simulink model "wlan_mac_dcf_hw"  (Simulink 7.8)
settings: Solver=ode45  StartTime=0.0  StopTime=1e5  RelTol=1e-3
PostLoadFcn:
  | wlan_mac_hw_init
InitFcn:
  | wlan_mac_hw_init
StartFcn:
  | wlan_mac_hw_init
values from neighbouring files (symbols this model uses):
  ticks_per_usec = 10    [wlan_mac_hw_init.m]
undefined symbols (not defined in the file or in its folder): gcbh, xlBlockLoadCallback, xlGetNormalizedPeriod
libraries: xbsIndex_r4 x422, xbsEDKLib_r4 x1
(part 3 of 4)

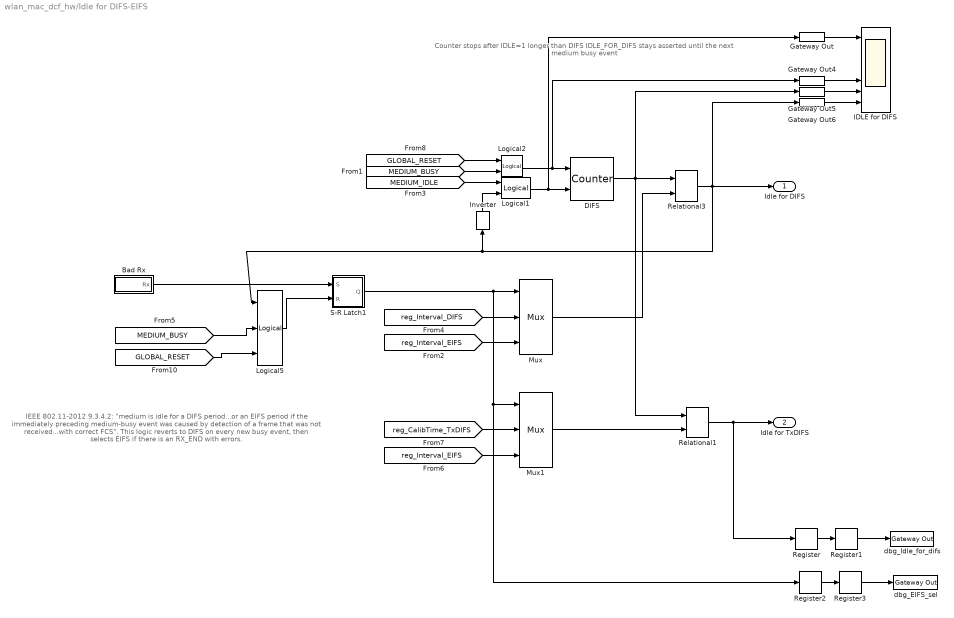
== system wlan_mac_dcf_hw/Idle for DIFS-EIFS ==
  note: IEEE 802.11-2012 9.3.4.2:
      | "medium is idle for a DIFS period...or an EIFS period if the immediately preceding medium-busy
      | event was caused by detection of a frame that was not received...with correct FCS".
      |
      | This logic reverts to DIFS on every new busy event, then
      | selects EIFS if there is an RX_END with errors.
  note: Counter stops after IDLE=1 longer than DIFS
      | IDLE_FOR_DIFS stays asserted until
      | the next medium busy event
  Bad Rx : Subsystem
  DIFS : xbsIndex_r4/Counter  cnt_type=Free Running  cnt_to=inf  operation=Up  start_count=0  cnt_by_val=1  arith_type=Unsigned  n_bits=NB_CNTR_DIFS  bin_pt=0  load_pin=off  rst=on  en=on  explicit_period=off  period=1  dbl_ovrd=off  use_behavioral_HDL=off  implementation=Fabric  block_type=counter
  Gateway Out{,4..6} (4 alike) : xbsIndex_r4/Gateway Out  inherit_from_input=off  hdl_port=off  timing_constraint=None  locs_specified=off  LOCs={}  UseAsDAC=off  DACChannel='1'  block_type=gatewayout
  IDLE for DIFS : Scope  NumInputPorts=7
      settings: YMin=-5~-5~-5~-5~-5~-5~-5  YMax=5~5~5~5~5~5~5  SaveName=ScopeData4
  Inverter : xbsIndex_r4/Inverter  en=off  latency=0  dbl_ovrd=off  block_type=inv
      settings: xl_area=[0 0 0 0 0 0 0]  block_version=VER_STRING_GOES_HERE
  Logical1 : xbsIndex_r4/Logical  logical_function=AND  inputs=2  en=off  latency=0  precision=Full  arith_type=Unsigned  n_bits=16  bin_pt=0  align_bp=on  dbl_ovrd=off  block_type=logical
  Logical2 : xbsIndex_r4/Logical  logical_function=OR  inputs=2  en=off  latency=0  precision=Full  arith_type=Unsigned  n_bits=8  bin_pt=2  align_bp=on  dbl_ovrd=off  block_type=logical
      settings: xl_area=[1 0 0 1 0 0 0]  block_version=VER_STRING_GOES_HERE
  Logical5 : xbsIndex_r4/Logical  logical_function=OR  inputs=3  en=off  latency=0  precision=Full  arith_type=Unsigned  n_bits=16  bin_pt=0  align_bp=on  dbl_ovrd=off  block_type=logical
  Mux : xbsIndex_r4/Mux  inputs=2  en=off  latency=0  precision=Full  arith_type=Unsigned  n_bits=16  bin_pt=14  quantization=Truncate  overflow=Wrap  dbl_ovrd=off  block_type=mux
  Mux1 : xbsIndex_r4/Mux  inputs=2  en=off  latency=0  precision=Full  arith_type=Unsigned  n_bits=16  bin_pt=14  quantization=Truncate  overflow=Wrap  dbl_ovrd=off  block_type=mux
  Register{,1..3} (4 alike) : xbsIndex_r4/Register  init=0  rst=off  en=off  dbl_ovrd=off  block_type=register
  Relational1 : xbsIndex_r4/Relational  mode=a>=b  en=off  latency=0  dbl_ovrd=off  block_type=relational
  Relational3 : xbsIndex_r4/Relational  mode=a>=b  en=off  latency=0  dbl_ovrd=off  block_type=relational
  S-R Latch1 : Subsystem
  dbg_EIFS_sel : xbsIndex_r4/Gateway Out  inherit_from_input=off  hdl_port=on  timing_constraint=None  locs_specified=off  LOCs={}  UseAsDAC=off  DACChannel='1'  block_type=gatewayout
  dbg_Idle_for_difs : xbsIndex_r4/Gateway Out  inherit_from_input=off  hdl_port=on  timing_constraint=None  locs_specified=off  LOCs={}  UseAsDAC=off  DACChannel='1'  block_type=gatewayout
  Idle for DIFS : Outport
  Idle for TxDIFS : Outport  Port=2
  wires:
  Relational3/1 -> Idle for DIFS/1, Inverter/1, Logical5/1, Gateway Out6/1
  Mux/1 -> Relational3/2
  DIFS/1 -> Relational3/1, Relational1/1, Gateway Out5/1
  Logical2/1 -> DIFS/1, Gateway Out4/1
  Logical1/1 -> DIFS/2, Gateway Out/1
  [MEDIUM_IDLE] -> Logical1/1
  [reg_Interval_DIFS] -> Mux/2
  [reg_Interval_EIFS] -> Mux/3
  S-R Latch1/1(Q) -> Mux/1, Mux1/1, Register2/1
  Bad Rx/1(Rx) -> S-R Latch1/1(S)
  Logical5/1 -> S-R Latch1/2(R)
  [MEDIUM_BUSY] -> Logical5/2
  [reg_CalibTime_TxDIFS] -> Mux1/2
  [reg_Interval_EIFS] -> Mux1/3
  Mux1/1 -> Relational1/2
  Relational1/1 -> Idle for TxDIFS/1, Register/1
  Inverter/1 -> Logical1/2
  Gateway Out/1 -> IDLE for DIFS/1
  Gateway Out4/1 -> IDLE for DIFS/5
  Gateway Out5/1 -> IDLE for DIFS/6
  Gateway Out6/1 -> IDLE for DIFS/7
  [GLOBAL_RESET] -> Logical5/3
  [MEDIUM_BUSY] -> Logical2/2
  [GLOBAL_RESET] -> Logical2/1
  Register/1 -> Register1/1
  Register1/1 -> dbg_Idle_for_difs/1
  Register2/1 -> Register3/1
  Register3/1 -> dbg_EIFS_sel/1

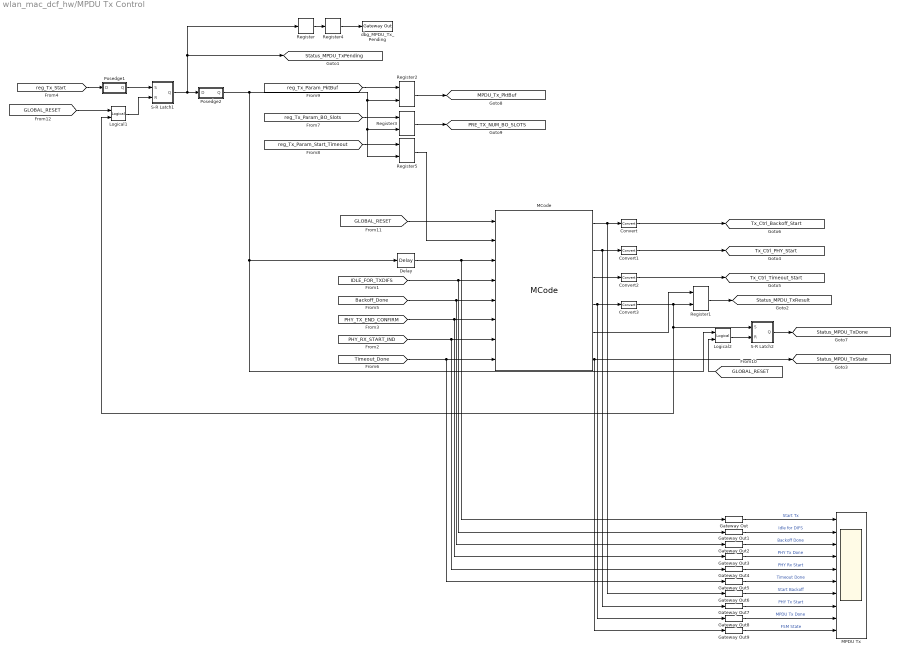
== system wlan_mac_dcf_hw/MPDU Tx Control ==
  Convert{,1..3} (4 alike) : xbsIndex_r4/Convert  gui_display_data_type=Boolean  arith_type=Boolean  n_bits=16  bin_pt=14  float_type=Single  exp_bits=8  fraction_bits=24  quantization=Truncate  overflow=Wrap  en=off  latency=0  dbl_ovrd=off  pipeline=off  block_type=convert
  Delay : xbsIndex_r4/Delay  rst=off  infoeditControl=Selection of Reset will increase slice count due to use of real FFs and instead of SRLs  en=off  latency=1  dbl_ovrd=off  reg_retiming=off  block_type=delay
  Gateway Out{,1..9} (10 alike) : xbsIndex_r4/Gateway Out  inherit_from_input=off  hdl_port=off  timing_constraint=None  locs_specified=off  LOCs={}  UseAsDAC=off  DACChannel='1'  block_type=gatewayout
  Logical1 : xbsIndex_r4/Logical  logical_function=OR  inputs=2  en=off  latency=0  precision=Full  arith_type=Unsigned  n_bits=8  bin_pt=2  align_bp=on  dbl_ovrd=off  block_type=logical
      settings: xl_area=[1 0 0 1 0 0 0]  block_version=VER_STRING_GOES_HERE
  Logical2 : xbsIndex_r4/Logical  logical_function=OR  inputs=2  en=off  latency=0  precision=Full  arith_type=Unsigned  n_bits=8  bin_pt=2  align_bp=on  dbl_ovrd=off  block_type=logical
      settings: xl_area=[1 0 0 1 0 0 0]  block_version=VER_STRING_GOES_HERE
  MCode : xbsIndex_r4/MCode  mfname=mac_tx_ctrl_fsm  explicit_period=on  period=1  inputsTable={'boundInpExpr'=>['','','','','','','',''],'inputs'=>['reset','timeout_req','new_tx','idle_for_difs','backoff_done','phy_tx_done','phy_rx_start','timeout_done']}  outputsTable={'outputs'=>['backoff_start','phy_tx_start','timeout_start','tx_done','tx_result_out','fsm_state_out'],'suppressOut'=>['off','off','off','off','off','off']}  dbl_ovrd=off  enable_stdout=off  enable_debug=off  suppress_output=on  defparams={}  hide_port_list={}  block_type=mcode
  MPDU Tx : Scope  NumInputPorts=10
      settings: YMin=-5~-5~-5~-5~-5~-5~-5~-5~-5~-5  YMax=5~5~5~5~5~5~5~5~5~5
  Posedge1 : Subsystem
  Posedge2 : Subsystem
  Register : xbsIndex_r4/Register  init=0  rst=off  en=off  dbl_ovrd=off  block_type=register
  Register{1..3,5} (4 alike) : xbsIndex_r4/Register  init=0  rst=off  en=on  dbl_ovrd=off  block_type=register
  Register4 : xbsIndex_r4/Register  init=0  rst=off  en=off  dbl_ovrd=off  block_type=register
  S-R Latch1 : Subsystem
  S-R Latch2 : Subsystem
  dbg_MPDU_Tx_Pending : xbsIndex_r4/Gateway Out  inherit_from_input=off  hdl_port=on  timing_constraint=None  locs_specified=off  LOCs={}  UseAsDAC=off  DACChannel='1'  block_type=gatewayout
  tag scope: MPDU_Tx_PktBuf=global, PRE_TX_NUM_BO_SLOTS=global, Status_MPDU_TxDone=global, Status_MPDU_TxPending=global, Status_MPDU_TxResult=global, Status_MPDU_TxState=global, Tx_Ctrl_Backoff_Start=global, Tx_Ctrl_PHY_Start=global, Tx_Ctrl_Timeout_Start=global
  wires:
  [reg_Tx_Param_BO_Slots] -> Register3/1
  [reg_Tx_Start] -> Posedge1/1(D)
  Posedge1/1(Q) -> S-R Latch1/1(S)
  S-R Latch1/1(Q) -> Posedge2/1(D), [Status_MPDU_TxPending], Register/1
  Posedge2/1(Q) -> Register3/2, Register5/2, Register2/2, Delay/1, Logical2/1
  Register3/1 -> [PRE_TX_NUM_BO_SLOTS]
  [reg_Tx_Param_PktBuf] -> Register2/1
  Register2/1 -> [MPDU_Tx_PktBuf]
  [reg_Tx_Param_Start_Timeout] -> Register5/1
  Delay/1 -> MCode/3, Gateway Out/1
  Register5/1 -> MCode/2
  [IDLE_FOR_TXDIFS] -> MCode/4, Gateway Out1/1
  [Backoff_Done] -> MCode/5, Gateway Out2/1
  [PHY_TX_END_CONFIRM] -> MCode/6, Gateway Out3/1
  [PHY_RX_START_IND] -> MCode/7, Gateway Out4/1
  [Timeout_Done] -> MCode/8, Gateway Out5/1
  [GLOBAL_RESET] -> MCode/1
  Logical1/1 -> S-R Latch1/2(R)
  [GLOBAL_RESET] -> Logical1/1
  MCode/4 -> Convert3/1, Gateway Out8/1
  MCode/2 -> Convert1/1, Gateway Out7/1
  MCode/3 -> Convert2/1
  MCode/1 -> Convert/1, Gateway Out6/1
  MCode/5 -> Register1/1
  Register1/1 -> [Status_MPDU_TxResult]
  MCode/6 -> [Status_MPDU_TxState], Gateway Out9/1
  S-R Latch2/1(Q) -> [Status_MPDU_TxDone]
  Convert/1 -> [Tx_Ctrl_Backoff_Start]
  Convert1/1 -> [Tx_Ctrl_PHY_Start]
  Convert2/1 -> [Tx_Ctrl_Timeout_Start]
  Convert3/1 -> Register1/2, S-R Latch2/1(S), Logical1/2
  Logical2/1 -> S-R Latch2/2(R)
  [GLOBAL_RESET] -> Logical2/2
  Gateway Out/1 -> MPDU Tx/1  "Start Tx"
  Gateway Out1/1 -> MPDU Tx/2  "Idle for DIFS"
  Gateway Out2/1 -> MPDU Tx/3  "Backoff Done"
  Gateway Out3/1 -> MPDU Tx/4  "PHY Tx Done"
  Gateway Out4/1 -> MPDU Tx/5  "PHY Rx Start"
  Gateway Out5/1 -> MPDU Tx/6  "Timeout Done"
  Gateway Out6/1 -> MPDU Tx/7  "Start Backoff"
  Gateway Out7/1 -> MPDU Tx/8  "PHY Tx Start"
  Gateway Out8/1 -> MPDU Tx/9  "MPDU Tx Done"
  Gateway Out9/1 -> MPDU Tx/10  "FSM State"
  Register/1 -> Register4/1
  Register4/1 -> dbg_MPDU_Tx_Pending/1

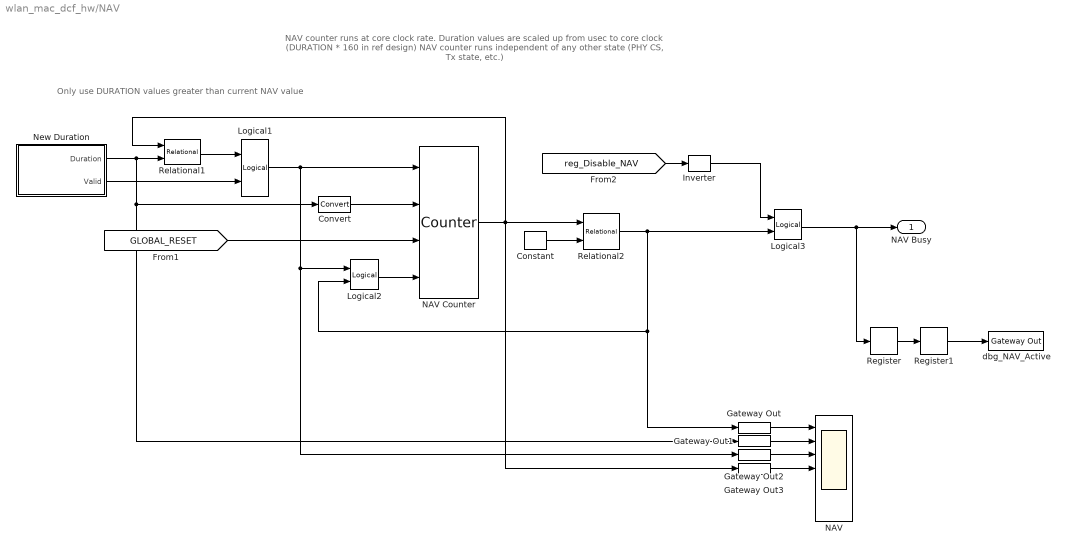
== system wlan_mac_dcf_hw/NAV ==
  note: NAV counter runs at core clock rate. Duration
      | values are scaled up from usec to core clock
      | (DURATION * 160 in ref design)
      |
      | NAV counter runs independent of any
      | other state (PHY CS, Tx state, etc.)
  note: Only use DURATION values greater
      | than current NAV value
  Constant : xbsIndex_r4/Constant  const=0  gui_display_data_type=Fixed-point  arith_type=Unsigned  n_bits=1  bin_pt=0  preci_type=Single  exp_width=8  frac_width=24  explicit_period=off  period=1  equ=P=C  opselect=C  inp2=PCIN>>17  opr=+  inp1=P  carry=CIN  dbl_ovrd=off  block_type=constant
  Convert : xbsIndex_r4/Convert  gui_display_data_type=Fixed-point  arith_type=Unsigned  n_bits=NB_CNTR_NAV  bin_pt=0  float_type=Single  exp_bits=8  fraction_bits=24  quantization=Truncate  overflow=Wrap  en=off  latency=0  dbl_ovrd=off  pipeline=off  block_type=convert
  Gateway Out{,1..3} (4 alike) : xbsIndex_r4/Gateway Out  inherit_from_input=off  hdl_port=off  timing_constraint=None  locs_specified=off  LOCs={}  UseAsDAC=off  DACChannel='1'  block_type=gatewayout
  Inverter : xbsIndex_r4/Inverter  en=off  latency=0  dbl_ovrd=off  block_type=inv
      settings: xl_area=[0 0 0 0 0 0 0]  block_version=VER_STRING_GOES_HERE
  Logical1 : xbsIndex_r4/Logical  logical_function=AND  inputs=2  en=off  latency=0  precision=Full  arith_type=Unsigned  n_bits=16  bin_pt=0  align_bp=on  dbl_ovrd=off  block_type=logical
  Logical2 : xbsIndex_r4/Logical  logical_function=OR  inputs=2  en=off  latency=0  precision=Full  arith_type=Unsigned  n_bits=16  bin_pt=0  align_bp=on  dbl_ovrd=off  block_type=logical
  Logical3 : xbsIndex_r4/Logical  logical_function=AND  inputs=2  en=off  latency=0  precision=Full  arith_type=Unsigned  n_bits=16  bin_pt=0  align_bp=on  dbl_ovrd=off  block_type=logical
  NAV : Scope  NumInputPorts=7
      settings: YMin=-5~-5~-5~-5~-5~-5~-5  YMax=5~5~5~5~5~5~5  SaveName=ScopeData3
  NAV Counter : xbsIndex_r4/Counter  cnt_type=Free Running  cnt_to=Inf  operation=Down  start_count=0  cnt_by_val=1  arith_type=Unsigned  n_bits=NB_CNTR_NAV  bin_pt=0  load_pin=on  rst=on  en=on  explicit_period=on  period=1  dbl_ovrd=off  use_behavioral_HDL=off  implementation=Fabric  block_type=counter
  New Duration : Subsystem
  Register : xbsIndex_r4/Register  init=0  rst=off  en=off  dbl_ovrd=off  block_type=register
  Register1 : xbsIndex_r4/Register  init=0  rst=off  en=off  dbl_ovrd=off  block_type=register
  Relational1 : xbsIndex_r4/Relational  mode=a<b  en=off  latency=0  dbl_ovrd=off  block_type=relational
  Relational2 : xbsIndex_r4/Relational  mode=a>b  en=off  latency=0  dbl_ovrd=off  block_type=relational
  dbg_NAV_Active : xbsIndex_r4/Gateway Out  inherit_from_input=off  hdl_port=on  timing_constraint=None  locs_specified=off  LOCs={}  UseAsDAC=off  DACChannel='1'  block_type=gatewayout
  NAV Busy : Outport
  wires:
  Logical1/1 -> NAV Counter/1, Logical2/1, Gateway Out2/1
  New Duration/2(Valid) -> Logical1/2
  NAV Counter/1 -> Relational2/1, Relational1/1, Gateway Out3/1
  [GLOBAL_RESET] -> NAV Counter/3
  Constant/1 -> Relational2/2
  Relational2/1 -> Gateway Out/1, Logical2/2, Logical3/2
  New Duration/1(Duration) -> Relational1/2, Convert/1, Gateway Out1/1
  Relational1/1 -> Logical1/1
  Convert/1 -> NAV Counter/2
  Gateway Out/1 -> NAV/1
  Gateway Out1/1 -> NAV/2
  Gateway Out2/1 -> NAV/3
  Gateway Out3/1 -> NAV/4
  Logical2/1 -> NAV Counter/4
  Logical3/1 -> NAV Busy/1, Register/1
  [reg_Disable_NAV] -> Inverter/1
  Inverter/1 -> Logical3/1
  Register/1 -> Register1/1
  Register1/1 -> dbg_NAV_Active/1

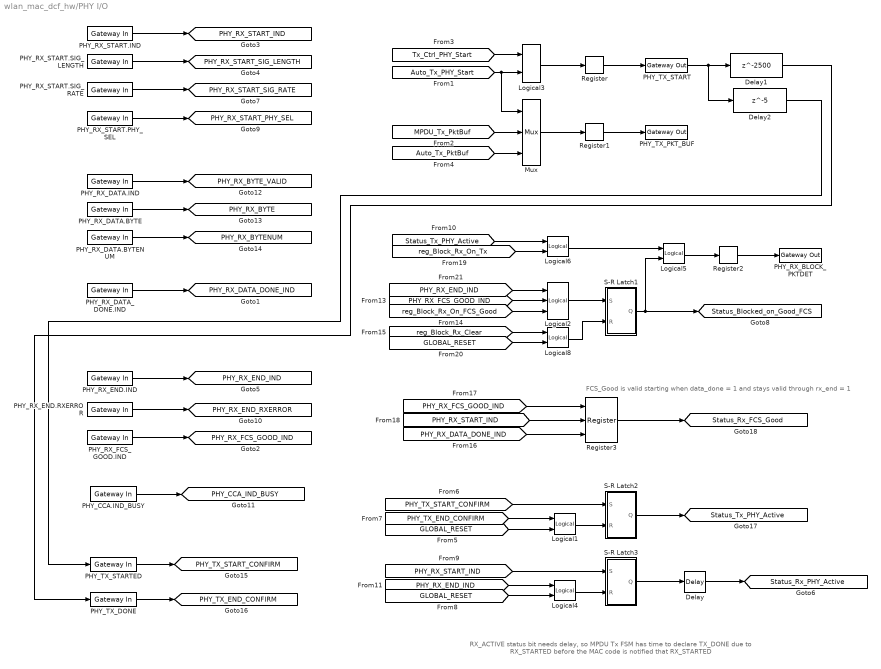
== system wlan_mac_dcf_hw/PHY I/O ==
  note: FCS_Good is valid starting when
      | data_done = 1 and stays valid through
      | rx_end = 1
  note: RX_ACTIVE status bit needs delay, so MPDU Tx FSM has time to declare TX_DONE
      |   due to RX_STARTED before the MAC code is notified that RX_STARTED
  Delay : xbsIndex_r4/Delay  rst=off  infoeditControl=Selection of Reset will increase slice count due to use of real FFs and instead of SRLs  en=off  latency=3  dbl_ovrd=off  reg_retiming=off  block_type=delay
  Delay1 : Delay  DelayLength=2500
  Delay2 : Delay  DelayLength=5
  Logical{1,4..5,8} (4 alike) : xbsIndex_r4/Logical  logical_function=OR  inputs=2  en=off  latency=0  precision=Full  arith_type=Unsigned  n_bits=8  bin_pt=2  align_bp=on  dbl_ovrd=off  block_type=logical
      settings: xl_area=[1 0 0 1 0 0 0]  block_version=VER_STRING_GOES_HERE
  Logical2 : xbsIndex_r4/Logical  logical_function=AND  inputs=3  en=off  latency=0  precision=Full  arith_type=Unsigned  n_bits=8  bin_pt=2  align_bp=on  dbl_ovrd=off  block_type=logical
      settings: xl_area=[1 0 0 1 0 0 0]  block_version=VER_STRING_GOES_HERE
  Logical3 : xbsIndex_r4/Logical  logical_function=OR  inputs=2  en=off  latency=0  precision=Full  arith_type=Unsigned  n_bits=16  bin_pt=0  align_bp=on  dbl_ovrd=off  block_type=logical
  Logical6 : xbsIndex_r4/Logical  logical_function=AND  inputs=2  en=off  latency=0  precision=Full  arith_type=Unsigned  n_bits=8  bin_pt=2  align_bp=on  dbl_ovrd=off  block_type=logical
      settings: xl_area=[1 0 0 1 0 0 0]  block_version=VER_STRING_GOES_HERE
  Mux : xbsIndex_r4/Mux  inputs=2  en=off  latency=0  precision=Full  arith_type=Unsigned  n_bits=16  bin_pt=14  quantization=Truncate  overflow=Wrap  dbl_ovrd=off  block_type=mux
  PHY_CCA.IND_BUSY : xbsIndex_r4/Gateway In  gui_display_data_type=Boolean  arith_type=Boolean  n_bits=16  bin_pt=14  preci_type=Single  exp_width=8  frac_width=24  quantization="Round  (unbiased: +/- Inf)"  overflow=Saturate  period=1  dbl_ovrd=off  timing_constraint=None  locs_specified=off  LOCs={}  UseAsADC=off  ADCChannel='1'  inherit_from_input=off  hdl_port=on  block_type=gatewayin
  PHY_RX_BLOCK_PKTDET : xbsIndex_r4/Gateway Out  inherit_from_input=off  hdl_port=on  timing_constraint=None  locs_specified=off  LOCs={}  UseAsDAC=off  DACChannel='1'  block_type=gatewayout
  PHY_RX_DATA.BYTE : xbsIndex_r4/Gateway In  gui_display_data_type=Fixed-point  arith_type=Unsigned  n_bits=8  bin_pt=0  preci_type=Single  exp_width=8  frac_width=24  quantization="Round  (unbiased: +/- Inf)"  overflow=Saturate  period=1  dbl_ovrd=off  timing_constraint=None  locs_specified=off  LOCs={}  UseAsADC=off  ADCChannel='1'  inherit_from_input=off  hdl_port=on  block_type=gatewayin
  PHY_RX_DATA.BYTENUM : xbsIndex_r4/Gateway In  gui_display_data_type=Fixed-point  arith_type=Unsigned  n_bits=14  bin_pt=0  preci_type=Single  exp_width=8  frac_width=24  quantization="Round  (unbiased: +/- Inf)"  overflow=Saturate  period=1  dbl_ovrd=off  timing_constraint=None  locs_specified=off  LOCs={}  UseAsADC=off  ADCChannel='1'  inherit_from_input=off  hdl_port=on  block_type=gatewayin
  PHY_RX_DATA.IND : xbsIndex_r4/Gateway In  gui_display_data_type=Boolean  arith_type=Boolean  n_bits=16  bin_pt=14  preci_type=Single  exp_width=8  frac_width=24  quantization="Round  (unbiased: +/- Inf)"  overflow=Saturate  period=1  dbl_ovrd=off  timing_constraint=None  locs_specified=off  LOCs={}  UseAsADC=off  ADCChannel='1'  inherit_from_input=off  hdl_port=on  block_type=gatewayin
  PHY_RX_DATA_DONE.IND : xbsIndex_r4/Gateway In  gui_display_data_type=Boolean  arith_type=Boolean  n_bits=1  bin_pt=0  preci_type=Single  exp_width=8  frac_width=24  quantization="Round  (unbiased: +/- Inf)"  overflow=Saturate  period=1  dbl_ovrd=off  timing_constraint=None  locs_specified=off  LOCs={}  UseAsADC=off  ADCChannel='1'  inherit_from_input=off  hdl_port=on  block_type=gatewayin
  PHY_RX_END.IND : xbsIndex_r4/Gateway In  gui_display_data_type=Boolean  arith_type=Boolean  n_bits=16  bin_pt=14  preci_type=Single  exp_width=8  frac_width=24  quantization="Round  (unbiased: +/- Inf)"  overflow=Saturate  period=1  dbl_ovrd=off  timing_constraint=None  locs_specified=off  LOCs={}  UseAsADC=off  ADCChannel='1'  inherit_from_input=off  hdl_port=on  block_type=gatewayin
  PHY_RX_END.RXERROR : xbsIndex_r4/Gateway In  gui_display_data_type=Fixed-point  arith_type=Unsigned  n_bits=2  bin_pt=0  preci_type=Single  exp_width=8  frac_width=24  quantization="Round  (unbiased: +/- Inf)"  overflow=Saturate  period=1  dbl_ovrd=off  timing_constraint=None  locs_specified=off  LOCs={}  UseAsADC=off  ADCChannel='1'  inherit_from_input=off  hdl_port=on  block_type=gatewayin
  PHY_RX_FCS_GOOD.IND : xbsIndex_r4/Gateway In  gui_display_data_type=Boolean  arith_type=Boolean  n_bits=1  bin_pt=0  preci_type=Single  exp_width=8  frac_width=24  quantization="Round  (unbiased: +/- Inf)"  overflow=Saturate  period=1  dbl_ovrd=off  timing_constraint=None  locs_specified=off  LOCs={}  UseAsADC=off  ADCChannel='1'  inherit_from_input=off  hdl_port=on  block_type=gatewayin
  PHY_RX_START.IND : xbsIndex_r4/Gateway In  gui_display_data_type=Boolean  arith_type=Boolean  n_bits=16  bin_pt=14  preci_type=Single  exp_width=8  frac_width=24  quantization="Round  (unbiased: +/- Inf)"  overflow=Saturate  period=1  dbl_ovrd=off  timing_constraint=None  locs_specified=off  LOCs={}  UseAsADC=off  ADCChannel='1'  inherit_from_input=off  hdl_port=on  block_type=gatewayin
  PHY_RX_START.PHY_SEL : xbsIndex_r4/Gateway In  gui_display_data_type=Boolean  arith_type=Boolean  n_bits=16  bin_pt=14  preci_type=Single  exp_width=8  frac_width=24  quantization="Round  (unbiased: +/- Inf)"  overflow=Saturate  period=1  dbl_ovrd=off  timing_constraint=None  locs_specified=off  LOCs={}  UseAsADC=off  ADCChannel='1'  inherit_from_input=off  hdl_port=on  block_type=gatewayin
  PHY_RX_START.SIG_LENGTH : xbsIndex_r4/Gateway In  gui_display_data_type=Fixed-point  arith_type=Unsigned  n_bits=12  bin_pt=0  preci_type=Single  exp_width=8  frac_width=24  quantization="Round  (unbiased: +/- Inf)"  overflow=Saturate  period=1  dbl_ovrd=off  timing_constraint=None  locs_specified=off  LOCs={}  UseAsADC=off  ADCChannel='1'  inherit_from_input=off  hdl_port=on  block_type=gatewayin
  PHY_RX_START.SIG_RATE : xbsIndex_r4/Gateway In  gui_display_data_type=Fixed-point  arith_type=Unsigned  n_bits=4  bin_pt=0  preci_type=Single  exp_width=8  frac_width=24  quantization="Round  (unbiased: +/- Inf)"  overflow=Saturate  period=1  dbl_ovrd=off  timing_constraint=None  locs_specified=off  LOCs={}  UseAsADC=off  ADCChannel='1'  inherit_from_input=off  hdl_port=on  block_type=gatewayin
  PHY_TX_DONE : xbsIndex_r4/Gateway In  gui_display_data_type=Boolean  arith_type=Boolean  n_bits=16  bin_pt=14  preci_type=Single  exp_width=8  frac_width=24  quantization="Round  (unbiased: +/- Inf)"  overflow=Saturate  period=1  dbl_ovrd=off  timing_constraint=None  locs_specified=off  LOCs={}  UseAsADC=off  ADCChannel='1'  inherit_from_input=off  hdl_port=on  block_type=gatewayin
  PHY_TX_PKT_BUF : xbsIndex_r4/Gateway Out  inherit_from_input=off  hdl_port=on  timing_constraint=None  locs_specified=off  LOCs={}  UseAsDAC=off  DACChannel='1'  block_type=gatewayout
  PHY_TX_START : xbsIndex_r4/Gateway Out  inherit_from_input=off  hdl_port=on  timing_constraint=None  locs_specified=off  LOCs={}  UseAsDAC=off  DACChannel='1'  block_type=gatewayout
  PHY_TX_STARTED : xbsIndex_r4/Gateway In  gui_display_data_type=Boolean  arith_type=Boolean  n_bits=16  bin_pt=14  preci_type=Single  exp_width=8  frac_width=24  quantization="Round  (unbiased: +/- Inf)"  overflow=Saturate  period=1  dbl_ovrd=off  timing_constraint=None  locs_specified=off  LOCs={}  UseAsADC=off  ADCChannel='1'  inherit_from_input=off  hdl_port=on  block_type=gatewayin
  Register : xbsIndex_r4/Register  init=0  rst=off  en=off  dbl_ovrd=off  block_type=register
  Register1 : xbsIndex_r4/Register  init=0  rst=off  en=off  dbl_ovrd=off  block_type=register
  Register2 : xbsIndex_r4/Register  init=0  rst=off  en=off  dbl_ovrd=off  block_type=register
  Register3 : xbsIndex_r4/Register  init=0  rst=on  en=on  dbl_ovrd=off  block_type=register
  S-R Latch1 : Subsystem
  S-R Latch2 : Subsystem
  S-R Latch3 : Subsystem
  tag scope: PHY_CCA_IND_BUSY=global, PHY_RX_BYTE=global, PHY_RX_BYTENUM=global, PHY_RX_BYTE_VALID=global, PHY_RX_DATA_DONE_IND=global, PHY_RX_END_IND=global, PHY_RX_END_RXERROR=global, PHY_RX_FCS_GOOD_IND=global, PHY_RX_START_IND=global, PHY_RX_START_PHY_SEL=global, PHY_RX_START_SIG_LENGTH=global, PHY_RX_START_SIG_RATE=global, PHY_TX_END_CONFIRM=global, PHY_TX_START_CONFIRM=global, Status_Blocked_on_Good_FCS=global, Status_Rx_FCS_Good=global, Status_Rx_PHY_Active=global, Status_Tx_PHY_Active=global
  wires:
  PHY_RX_DATA_DONE.IND/1 -> [PHY_RX_DATA_DONE_IND]
  PHY_RX_FCS_GOOD.IND/1 -> [PHY_RX_FCS_GOOD_IND]
  PHY_RX_START.IND/1 -> [PHY_RX_START_IND]
  PHY_RX_START.SIG_LENGTH/1 -> [PHY_RX_START_SIG_LENGTH]
  PHY_RX_END.IND/1 -> [PHY_RX_END_IND]
  PHY_RX_END.RXERROR/1 -> [PHY_RX_END_RXERROR]
  PHY_CCA.IND_BUSY/1 -> [PHY_CCA_IND_BUSY]
  PHY_RX_DATA.IND/1 -> [PHY_RX_BYTE_VALID]
  PHY_RX_DATA.BYTE/1 -> [PHY_RX_BYTE]
  PHY_RX_DATA.BYTENUM/1 -> [PHY_RX_BYTENUM]
  PHY_TX_STARTED/1 -> [PHY_TX_START_CONFIRM]
  PHY_TX_DONE/1 -> [PHY_TX_END_CONFIRM]
  Logical3/1 -> Register/1
  [Tx_Ctrl_PHY_Start] -> Logical3/1
  [Auto_Tx_PHY_Start] -> Logical3/2, Mux/1
  Mux/1 -> Register1/1
  [MPDU_Tx_PktBuf] -> Mux/2
  [Auto_Tx_PktBuf] -> Mux/3
  Register/1 -> PHY_TX_START/1
  Register1/1 -> PHY_TX_PKT_BUF/1
  [PHY_TX_START_CONFIRM] -> S-R Latch2/1(S)
  Logical1/1 -> S-R Latch2/2(R)
  [PHY_TX_END_CONFIRM] -> Logical1/1
  [GLOBAL_RESET] -> Logical1/2
  S-R Latch2/1(Q) -> [Status_Tx_PHY_Active]
  [PHY_RX_START_IND] -> S-R Latch3/1(S)
  Logical4/1 -> S-R Latch3/2(R)
  [PHY_RX_END_IND] -> Logical4/1
  [GLOBAL_RESET] -> Logical4/2
  S-R Latch3/1(Q) -> Delay/1
  Register2/1 -> PHY_RX_BLOCK_PKTDET/1
  Logical6/1 -> Logical5/1
  [PHY_RX_END_IND] -> Logical2/1
  [PHY_RX_FCS_GOOD_IND] -> Logical2/2
  [reg_Block_Rx_On_FCS_Good] -> Logical2/3
  Logical2/1 -> S-R Latch1/1(S)
  S-R Latch1/1(Q) -> Logical5/2, [Status_Blocked_on_Good_FCS]
  Logical5/1 -> Register2/1
  PHY_RX_START.SIG_RATE/1 -> [PHY_RX_START_SIG_RATE]
  PHY_RX_START.PHY_SEL/1 -> [PHY_RX_START_PHY_SEL]
  Logical8/1 -> S-R Latch1/2(R)
  [reg_Block_Rx_Clear] -> Logical8/1
  [GLOBAL_RESET] -> Logical8/2
  [PHY_RX_FCS_GOOD_IND] -> Register3/1
  Register3/1 -> [Status_Rx_FCS_Good]
  [PHY_RX_DATA_DONE_IND] -> Register3/3
  [PHY_RX_START_IND] -> Register3/2
  [Status_Tx_PHY_Active] -> Logical6/1
  [reg_Block_Rx_On_Tx] -> Logical6/2
  Delay/1 -> [Status_Rx_PHY_Active]
  PHY_TX_START/1 -> Delay1/1, Delay2/1
  Delay1/1 -> PHY_TX_DONE/1
  Delay2/1 -> PHY_TX_STARTED/1

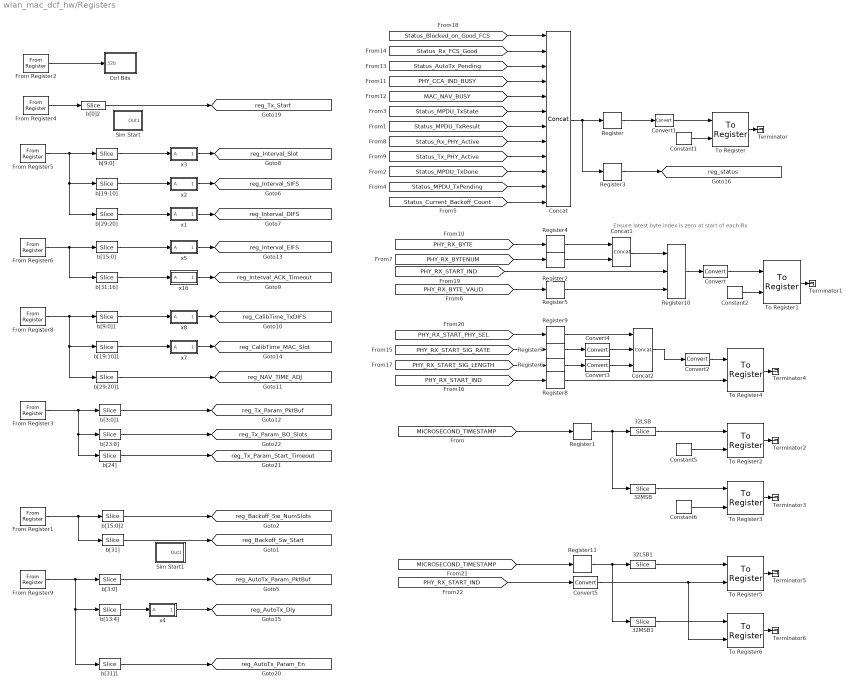
== system wlan_mac_dcf_hw/Registers ==
  note: Ensure latest byte index is zero
      | at start of each Rx
  " b[13:4]" : xbsIndex_r4/Slice  nbits=10  boolean_output=off  mode=Lower Bit Location + Width  bit1=0  base1=MSB of Input  bit0=4  base0=LSB of Input  dbl_ovrd=off  block_type=slice
      settings: block_version=VER_STRING_GOES_HERE
  " b[15:0]" : xbsIndex_r4/Slice  nbits=16  boolean_output=off  mode=Lower Bit Location + Width  bit1=0  base1=MSB of Input  bit0=0  base0=LSB of Input  dbl_ovrd=off  block_type=slice
      settings: block_version=VER_STRING_GOES_HERE
  " b[15:0]2" : xbsIndex_r4/Slice  nbits=16  boolean_output=off  mode=Lower Bit Location + Width  bit1=0  base1=MSB of Input  bit0=0  base0=LSB of Input  dbl_ovrd=off  block_type=slice
      settings: block_version=VER_STRING_GOES_HERE
  " b[19:10]" : xbsIndex_r4/Slice  nbits=10  boolean_output=off  mode=Lower Bit Location + Width  bit1=0  base1=MSB of Input  bit0=10  base0=LSB of Input  dbl_ovrd=off  block_type=slice
      settings: block_version=VER_STRING_GOES_HERE
  " b[19:10]1" : xbsIndex_r4/Slice  nbits=10  boolean_output=off  mode=Lower Bit Location + Width  bit1=0  base1=MSB of Input  bit0=10  base0=LSB of Input  dbl_ovrd=off  block_type=slice
      settings: block_version=VER_STRING_GOES_HERE
  " b[23:8]" : xbsIndex_r4/Slice  nbits=16  boolean_output=off  mode=Lower Bit Location + Width  bit1=0  base1=MSB of Input  bit0=8  base0=LSB of Input  dbl_ovrd=off  block_type=slice
      settings: block_version=VER_STRING_GOES_HERE
  " b[24]" : xbsIndex_r4/Slice  nbits=1  boolean_output=on  mode=Lower Bit Location + Width  bit1=0  base1=MSB of Input  bit0=24  base0=LSB of Input  dbl_ovrd=off  block_type=slice
      settings: block_version=VER_STRING_GOES_HERE
  " b[29:20]" : xbsIndex_r4/Slice  nbits=10  boolean_output=off  mode=Lower Bit Location + Width  bit1=0  base1=MSB of Input  bit0=20  base0=LSB of Input  dbl_ovrd=off  block_type=slice
      settings: block_version=VER_STRING_GOES_HERE
  " b[29:20]1" : xbsIndex_r4/Slice  nbits=10  boolean_output=off  mode=Lower Bit Location + Width  bit1=0  base1=MSB of Input  bit0=20  base0=LSB of Input  dbl_ovrd=off  block_type=slice
      settings: block_version=VER_STRING_GOES_HERE
  " b[31:16]" : xbsIndex_r4/Slice  nbits=16  boolean_output=off  mode=Lower Bit Location + Width  bit1=0  base1=MSB of Input  bit0=16  base0=LSB of Input  dbl_ovrd=off  block_type=slice
      settings: block_version=VER_STRING_GOES_HERE
  " b[31]" : xbsIndex_r4/Slice  nbits=1  boolean_output=on  mode=Lower Bit Location + Width  bit1=0  base1=MSB of Input  bit0=31  base0=LSB of Input  dbl_ovrd=off  block_type=slice
      settings: block_version=VER_STRING_GOES_HERE
  " b[31]1" : xbsIndex_r4/Slice  nbits=1  boolean_output=on  mode=Lower Bit Location + Width  bit1=0  base1=MSB of Input  bit0=31  base0=LSB of Input  dbl_ovrd=off  block_type=slice
      settings: block_version=VER_STRING_GOES_HERE
  " b[3:0]" : xbsIndex_r4/Slice  nbits=4  boolean_output=off  mode=Lower Bit Location + Width  bit1=0  base1=MSB of Input  bit0=0  base0=LSB of Input  dbl_ovrd=off  block_type=slice
      settings: block_version=VER_STRING_GOES_HERE
  " b[3:0]1" : xbsIndex_r4/Slice  nbits=4  boolean_output=off  mode=Lower Bit Location + Width  bit1=0  base1=MSB of Input  bit0=0  base0=LSB of Input  dbl_ovrd=off  block_type=slice
      settings: block_version=VER_STRING_GOES_HERE
  " b[9:0]" : xbsIndex_r4/Slice  nbits=10  boolean_output=off  mode=Lower Bit Location + Width  bit1=0  base1=MSB of Input  bit0=0  base0=LSB of Input  dbl_ovrd=off  block_type=slice
      settings: block_version=VER_STRING_GOES_HERE
  " b[9:0]1" : xbsIndex_r4/Slice  nbits=10  boolean_output=off  mode=Lower Bit Location + Width  bit1=0  base1=MSB of Input  bit0=0  base0=LSB of Input  dbl_ovrd=off  block_type=slice
      settings: block_version=VER_STRING_GOES_HERE
  32LSB : xbsIndex_r4/Slice  nbits=32  boolean_output=off  mode=Lower Bit Location + Width  bit1=0  base1=MSB of Input  bit0=0  base0=LSB of Input  dbl_ovrd=off  block_type=slice
      settings: block_version=VER_STRING_GOES_HERE
  32LSB1 : xbsIndex_r4/Slice  nbits=32  boolean_output=off  mode=Lower Bit Location + Width  bit1=0  base1=MSB of Input  bit0=0  base0=LSB of Input  dbl_ovrd=off  block_type=slice
      settings: block_version=VER_STRING_GOES_HERE
  32MSB : xbsIndex_r4/Slice  nbits=32  boolean_output=off  mode=Upper Bit Location + Width  bit1=0  base1=MSB of Input  bit0=0  base0=LSB of Input  dbl_ovrd=off  block_type=slice
      settings: block_version=VER_STRING_GOES_HERE
  32MSB1 : xbsIndex_r4/Slice  nbits=32  boolean_output=off  mode=Upper Bit Location + Width  bit1=0  base1=MSB of Input  bit0=0  base0=LSB of Input  dbl_ovrd=off  block_type=slice
      settings: block_version=VER_STRING_GOES_HERE
  Concat : xbsIndex_r4/Concat  num_inputs=12  dbl_ovrd=off  block_type=concat
      settings: block_version=8.2.02
  Concat1 : xbsIndex_r4/Concat  num_inputs=2  dbl_ovrd=off  block_type=concat
      settings: block_version=8.2.02
  Concat2 : xbsIndex_r4/Concat  num_inputs=3  dbl_ovrd=off  block_type=concat
      settings: block_version=8.2.02
  Constant{1..2,5..6} (4 alike) : xbsIndex_r4/Constant  const=1  gui_display_data_type=Boolean  arith_type=Boolean  n_bits=30  bin_pt=0  preci_type=Single  exp_width=8  frac_width=24  explicit_period=on  period=1  equ=P=C  opselect=C  inp2=PCIN>>17  opr=+  inp1=P  carry=CIN  dbl_ovrd=off  block_type=constant
  Convert : xbsIndex_r4/Convert  gui_display_data_type=Fixed-point  arith_type=Unsigned  n_bits=32  bin_pt=0  float_type=Single  exp_bits=8  fraction_bits=24  quantization=Truncate  overflow=Wrap  en=off  latency=0  dbl_ovrd=off  pipeline=off  block_type=convert
  Convert1 : xbsIndex_r4/Convert  gui_display_data_type=Fixed-point  arith_type=Unsigned  n_bits=32  bin_pt=0  float_type=Single  exp_bits=8  fraction_bits=24  quantization=Truncate  overflow=Wrap  en=off  latency=0  dbl_ovrd=off  pipeline=off  block_type=convert
  Convert2 : xbsIndex_r4/Convert  gui_display_data_type=Fixed-point  arith_type=Unsigned  n_bits=32  bin_pt=0  float_type=Single  exp_bits=8  fraction_bits=24  quantization=Truncate  overflow=Wrap  en=off  latency=0  dbl_ovrd=off  pipeline=off  block_type=convert
  Convert3 : xbsIndex_r4/Convert  gui_display_data_type=Fixed-point  arith_type=Unsigned  n_bits=16  bin_pt=0  float_type=Single  exp_bits=8  fraction_bits=24  quantization=Truncate  overflow=Wrap  en=off  latency=0  dbl_ovrd=off  pipeline=off  block_type=convert
  Convert4 : xbsIndex_r4/Convert  gui_display_data_type=Fixed-point  arith_type=Unsigned  n_bits=8  bin_pt=0  float_type=Single  exp_bits=8  fraction_bits=24  quantization=Truncate  overflow=Wrap  en=off  latency=0  dbl_ovrd=off  pipeline=off  block_type=convert
  Convert5 : xbsIndex_r4/Convert  gui_display_data_type=Boolean  arith_type=Boolean  n_bits=32  bin_pt=0  float_type=Single  exp_bits=8  fraction_bits=24  quantization=Truncate  overflow=Wrap  en=off  latency=0  dbl_ovrd=off  pipeline=off  block_type=convert
  Ctrl Bits : Subsystem
  From Register1 : xbsIndex_r4/From Register  shared_memory_name='BACKOFF_CTRL'  init=REG_MAC_Backoff_Control  period=1  ownership=Locally owned and initialized  gui_display_data_type=Fixed-point  arith_type=Unsigned  n_bits=32  bin_pt=0  preci_type=Single  dbl_ovrd=off  block_type=fromreg
      settings: AttributesFormatString=<< %<shared_memory_name> >>  infoedit="Register block that reads data to a shared memory register.  Delay of one sample period."
  From Register2 : xbsIndex_r4/From Register  shared_memory_name='Control'  init=0  period=1  ownership=Locally owned and initialized  gui_display_data_type=Fixed-point  arith_type=Unsigned  n_bits=32  bin_pt=0  preci_type=Single  dbl_ovrd=off  block_type=fromreg
      settings: AttributesFormatString=<< %<shared_memory_name> >>  infoedit="Register block that reads data to a shared memory register.  Delay of one sample period."
  From Register3 : xbsIndex_r4/From Register  shared_memory_name='MPDU_TX_PARAMS'  init=REG_MAC_MPDU_Tx_Params  period=1  ownership=Locally owned and initialized  gui_display_data_type=Fixed-point  arith_type=Unsigned  n_bits=32  bin_pt=0  preci_type=Single  dbl_ovrd=off  block_type=fromreg
      settings: AttributesFormatString=<< %<shared_memory_name> >>  infoedit="Register block that reads data to a shared memory register.  Delay of one sample period."
  From Register4 : xbsIndex_r4/From Register  shared_memory_name='TX_START'  init=0  period=1  ownership=Locally owned and initialized  gui_display_data_type=Fixed-point  arith_type=Unsigned  n_bits=32  bin_pt=0  preci_type=Single  dbl_ovrd=off  block_type=fromreg
      settings: AttributesFormatString=<< %<shared_memory_name> >>  infoedit="Register block that reads data to a shared memory register.  Delay of one sample period."
  From Register5 : xbsIndex_r4/From Register  shared_memory_name='IFS_INTERVALS1'  init=REG_MAC_Intervals_1  period=1  ownership=Locally owned and initialized  gui_display_data_type=Fixed-point  arith_type=Unsigned  n_bits=32  bin_pt=0  preci_type=Single  dbl_ovrd=off  block_type=fromreg
      settings: AttributesFormatString=<< %<shared_memory_name> >>  infoedit="Register block that reads data to a shared memory register.  Delay of one sample period."
  From Register6 : xbsIndex_r4/From Register  shared_memory_name='IFS_INTERVALS2'  init=REG_MAC_Intervals_2  period=1  ownership=Locally owned and initialized  gui_display_data_type=Fixed-point  arith_type=Unsigned  n_bits=32  bin_pt=0  preci_type=Single  dbl_ovrd=off  block_type=fromreg
      settings: AttributesFormatString=<< %<shared_memory_name> >>  infoedit="Register block that reads data to a shared memory register.  Delay of one sample period."
  From Register8 : xbsIndex_r4/From Register  shared_memory_name='CALIB_TIMES'  init=REG_MAC_Calib_Times  period=1  ownership=Locally owned and initialized  gui_display_data_type=Fixed-point  arith_type=Unsigned  n_bits=32  bin_pt=0  preci_type=Single  dbl_ovrd=off  block_type=fromreg
      settings: AttributesFormatString=<< %<shared_memory_name> >>  infoedit="Register block that reads data to a shared memory register.  Delay of one sample period."
  From Register9 : xbsIndex_r4/From Register  shared_memory_name='AUTO_TX_PARAMS'  init=REG_MAC_Auto_Tx_Params  period=1  ownership=Locally owned and initialized  gui_display_data_type=Fixed-point  arith_type=Unsigned  n_bits=32  bin_pt=0  preci_type=Single  dbl_ovrd=off  block_type=fromreg
      settings: AttributesFormatString=<< %<shared_memory_name> >>  infoedit="Register block that reads data to a shared memory register.  Delay of one sample period."
  Register{,1..9,11} (11 alike) : xbsIndex_r4/Register  init=0  rst=off  en=off  dbl_ovrd=off  block_type=register
  Register10 : xbsIndex_r4/Register  init=0  rst=on  en=on  dbl_ovrd=off  block_type=register
  Sim Start : Subsystem
  Sim Start1 : Subsystem
  Terminator{,1..6} (7 alike) : Terminator
  To Register : xbsIndex_r4/To Register  shared_memory_name='Status'  init=0  ownership=Locally owned and initialized  explicit_data_type=on  gui_display_data_type=Fixed-point  arith_type=Unsigned  n_bits=32  bin_pt=0  preci_type=Single  dbl_ovrd=off  block_type=toreg
      settings: AttributesFormatString=<< %<shared_memory_name> >>  infoedit="Register block that writes data to a shared memory register.  Delay of one sample period."
  To Register1 : xbsIndex_r4/To Register  shared_memory_name='LATEST_RX_BYTE'  init=0  ownership=Locally owned and initialized  explicit_data_type=on  gui_display_data_type=Fixed-point  arith_type=Unsigned  n_bits=32  bin_pt=0  preci_type=Single  dbl_ovrd=off  block_type=toreg
      settings: AttributesFormatString=<< %<shared_memory_name> >>  infoedit="Register block that writes data to a shared memory register.  Delay of one sample period."
  To Register2 : xbsIndex_r4/To Register  shared_memory_name='TIMESTAMP_LSB'  init=0  ownership=Locally owned and initialized  explicit_data_type=on  gui_display_data_type=Fixed-point  arith_type=Unsigned  n_bits=32  bin_pt=0  preci_type=Single  dbl_ovrd=off  block_type=toreg
      settings: AttributesFormatString=<< %<shared_memory_name> >>  infoedit="Register block that writes data to a shared memory register.  Delay of one sample period."
  To Register3 : xbsIndex_r4/To Register  shared_memory_name='TIMESTAMP_MSB'  init=0  ownership=Locally owned and initialized  explicit_data_type=on  gui_display_data_type=Fixed-point  arith_type=Unsigned  n_bits=32  bin_pt=0  preci_type=Single  dbl_ovrd=off  block_type=toreg
      settings: AttributesFormatString=<< %<shared_memory_name> >>  infoedit="Register block that writes data to a shared memory register.  Delay of one sample period."
  To Register4 : xbsIndex_r4/To Register  shared_memory_name='RX_RATE_LENGTH'  init=0  ownership=Locally owned and initialized  explicit_data_type=on  gui_display_data_type=Fixed-point  arith_type=Unsigned  n_bits=32  bin_pt=0  preci_type=Single  dbl_ovrd=off  block_type=toreg
      settings: AttributesFormatString=<< %<shared_memory_name> >>  infoedit="Register block that writes data to a shared memory register.  Delay of one sample period."
  To Register5 : xbsIndex_r4/To Register  shared_memory_name='RX_START_TIMESTAMP_LSB'  init=0  ownership=Locally owned and initialized  explicit_data_type=on  gui_display_data_type=Fixed-point  arith_type=Unsigned  n_bits=32  bin_pt=0  preci_type=Single  dbl_ovrd=off  block_type=toreg
      settings: AttributesFormatString=<< %<shared_memory_name> >>  infoedit="Register block that writes data to a shared memory register.  Delay of one sample period."
  To Register6 : xbsIndex_r4/To Register  shared_memory_name='RX_START_TIMESTAMP_MSB'  init=0  ownership=Locally owned and initialized  explicit_data_type=on  gui_display_data_type=Fixed-point  arith_type=Unsigned  n_bits=32  bin_pt=0  preci_type=Single  dbl_ovrd=off  block_type=toreg
      settings: AttributesFormatString=<< %<shared_memory_name> >>  infoedit="Register block that writes data to a shared memory register.  Delay of one sample period."
  b[0]2 : xbsIndex_r4/Slice  nbits=1  boolean_output=on  mode=Lower Bit Location + Width  bit1=0  base1=MSB of Input  bit0=0  base0=LSB of Input  dbl_ovrd=off  block_type=slice
      settings: block_version=VER_STRING_GOES_HERE
  x1 : Subsystem
  x16 : Subsystem
  x2 : Subsystem
  x3 : Subsystem
  x4 : Subsystem
  x5 : Subsystem
  x7 : Subsystem
  x8 : Subsystem
  tag scope: reg_AutoTx_Dly=global, reg_AutoTx_Param_En=global, reg_AutoTx_Param_PktBuf=global, reg_Backoff_Sw_NumSlots=global, reg_Backoff_Sw_Start=global, reg_CalibTime_MAC_Slot=global, reg_CalibTime_TxDIFS=global, reg_Interval_ACK_Timeout=global, reg_Interval_DIFS=global, reg_Interval_EIFS=global, reg_Interval_SIFS=global, reg_Interval_Slot=global, reg_NAV_TIME_ADJ=global, reg_Tx_Param_BO_Slots=global, reg_Tx_Param_PktBuf=global, reg_Tx_Param_Start_Timeout=global, reg_Tx_Start=global, reg_status=global
  wires:
  From Register2/1 -> Ctrl Bits/1(32b)
  Constant1/1 -> To Register/2
  To Register/1 -> Terminator/1
  Concat/1 -> Register3/1, Register/1
  32LSB/1 -> To Register2/1
  Constant5/1 -> To Register2/2
  32MSB/1 -> To Register3/1
  Constant6/1 -> To Register3/2
  [MICROSECOND_TIMESTAMP] -> Register1/1
  x16/1(Ax16) -> [reg_Interval_ACK_Timeout]
  x1/1(Ax16) -> [reg_Interval_DIFS]
  x2/1(Ax16) -> [reg_Interval_SIFS]
  x3/1(Ax16) -> [reg_Interval_Slot]
  x5/1(Ax16) -> [reg_Interval_EIFS]
  From Register3/1 -> " b[23:8]"/1, " b[24]"/1, " b[3:0]1"/1
  b[0]2/1 -> [reg_Tx_Start]
  From Register5/1 -> " b[9:0]"/1, " b[19:10]"/1, " b[29:20]"/1
  From Register6/1 -> " b[15:0]"/1, " b[31:16]"/1
  " b[9:0]"/1 -> x3/1(A)
  " b[19:10]"/1 -> x2/1(A)
  " b[29:20]"/1 -> x1/1(A)
  " b[15:0]"/1 -> x5/1(A)
  " b[31:16]"/1 -> x16/1(A)
  x7/1(Ax16) -> [reg_CalibTime_MAC_Slot]
  x8/1(Ax16) -> [reg_CalibTime_TxDIFS]
  From Register8/1 -> " b[9:0]1"/1, " b[19:10]1"/1, " b[29:20]1"/1
  " b[9:0]1"/1 -> x8/1(A)
  " b[19:10]1"/1 -> x7/1(A)
  " b[29:20]1"/1 -> [reg_NAV_TIME_ADJ]
  " b[24]"/1 -> [reg_Tx_Param_Start_Timeout]
  From Register1/1 -> " b[15:0]2"/1, " b[31]"/1
  " b[15:0]2"/1 -> [reg_Backoff_Sw_NumSlots]
  " b[31]"/1 -> [reg_Backoff_Sw_Start]
  From Register9/1 -> " b[3:0]"/1, " b[31]1"/1, " b[13:4]"/1
  " b[3:0]"/1 -> [reg_AutoTx_Param_PktBuf]
  To Register1/1 -> Terminator1/1
  [PHY_RX_BYTE_VALID] -> Register5/1
  [PHY_RX_BYTENUM] -> Register2/1
  " b[3:0]1"/1 -> [reg_Tx_Param_PktBuf]
  " b[23:8]"/1 -> [reg_Tx_Param_BO_Slots]
  " b[31]1"/1 -> [reg_AutoTx_Param_En]
  " b[13:4]"/1 -> x4/1(A)
  x4/1(Ax16) -> [reg_AutoTx_Dly]
  Register/1 -> Convert1/1
  Register1/1 -> 32LSB/1, 32MSB/1
  Register2/1 -> Concat1/2
  Convert1/1 -> To Register/1
  Register3/1 -> [reg_status]
  Register4/1 -> Concat1/1
  Register5/1 -> Register10/3
  [PHY_RX_BYTE] -> Register4/1
  To Register2/1 -> Terminator2/1
  To Register3/1 -> Terminator3/1
  From Register4/1 -> b[0]2/1
  [PHY_CCA_IND_BUSY] -> Concat/4
  [MAC_NAV_BUSY] -> Concat/5
  [Status_MPDU_TxState] -> Concat/6
  [Status_MPDU_TxResult] -> Concat/7
  [Status_Rx_PHY_Active] -> Concat/8
  [Status_Tx_PHY_Active] -> Concat/9
  [Status_MPDU_TxDone] -> Concat/10
  [Status_MPDU_TxPending] -> Concat/11
  [Status_Current_Backoff_Count] -> Concat/12
  Concat1/1 -> Register10/1
  [Status_AutoTx_Pending] -> Concat/3
  [Status_Rx_FCS_Good] -> Concat/2
  To Register4/1 -> Terminator4/1
  [PHY_RX_START_SIG_LENGTH] -> Register6/1
  Register6/1 -> Convert3/1
  Register7/1 -> Convert4/1
  Register8/1 -> To Register4/2
  [PHY_RX_START_SIG_RATE] -> Register7/1
  Convert2/1 -> To Register4/1
  [PHY_RX_START_IND] -> Register8/1
  Convert3/1 -> Concat2/3
  [Status_Blocked_on_Good_FCS] -> Concat/1
  [PHY_RX_START_PHY_SEL] -> Register9/1
  Convert4/1 -> Concat2/2
  Register9/1 -> Concat2/1
  Concat2/1 -> Convert2/1
  Register10/1 -> Convert/1
  Convert/1 -> To Register1/1
  Constant2/1 -> To Register1/2
  [PHY_RX_START_IND] -> Register10/2
  32LSB1/1 -> To Register5/1
  [PHY_RX_START_IND] -> Convert5/1
  32MSB1/1 -> To Register6/1
  [MICROSECOND_TIMESTAMP] -> Register11/1
  Register11/1 -> 32MSB1/1, 32LSB1/1
  To Register5/1 -> Terminator5/1
  To Register6/1 -> Terminator6/1
  Convert5/1 -> To Register5/2, To Register6/2

== system wlan_mac_dcf_hw/Resets ==
  Convert1 : xbsIndex_r4/Convert  gui_display_data_type=Boolean  arith_type=Boolean  n_bits=16  bin_pt=14  float_type=Single  exp_bits=8  fraction_bits=24  quantization=Truncate  overflow=Wrap  en=off  latency=0  dbl_ovrd=off  pipeline=off  block_type=convert
  Convert2 : xbsIndex_r4/Convert  gui_display_data_type=Boolean  arith_type=Boolean  n_bits=16  bin_pt=14  float_type=Single  exp_bits=8  fraction_bits=24  quantization=Truncate  overflow=Wrap  en=off  latency=0  dbl_ovrd=off  pipeline=off  block_type=convert
  Logical : xbsIndex_r4/Logical  logical_function=OR  inputs=2  en=off  latency=0  precision=Full  arith_type=Unsigned  n_bits=16  bin_pt=0  align_bp=on  dbl_ovrd=off  block_type=logical
  Pulse Generator : DiscretePulseGenerator  Period=1e9  PulseWidth=8  PhaseDelay=10
  RESET : xbsIndex_r4/Gateway In  gui_display_data_type=Fixed-point  arith_type=Unsigned  n_bits=1  bin_pt=0  preci_type=Single  exp_width=8  frac_width=24  quantization=Truncate  overflow=Wrap  period=1  dbl_ovrd=off  timing_constraint=None  locs_specified=off  LOCs={}  UseAsADC=off  ADCChannel='1'  inherit_from_input=off  hdl_port=on  block_type=gatewayin
  tag scope: GLOBAL_RESET=global
  wires:
  [reg_Global_Reset] -> Convert1/1
  RESET/1 -> Convert2/1
  Pulse Generator/1 -> RESET/1
  Convert1/1 -> Logical/1
  Convert2/1 -> Logical/2
  Logical/1 -> [GLOBAL_RESET]

== system wlan_mac_dcf_hw/Timeout ==
  Inverter : xbsIndex_r4/Inverter  en=off  latency=0  dbl_ovrd=off  block_type=inv
      settings: xl_area=[0 0 0 0 0 0 0]  block_version=VER_STRING_GOES_HERE
  Logical2 : xbsIndex_r4/Logical  logical_function=OR  inputs=2  en=off  latency=0  precision=Full  arith_type=Unsigned  n_bits=8  bin_pt=2  align_bp=on  dbl_ovrd=off  block_type=logical
      settings: xl_area=[1 0 0 1 0 0 0]  block_version=VER_STRING_GOES_HERE
  Logical3 : xbsIndex_r4/Logical  logical_function=OR  inputs=3  en=off  latency=0  precision=Full  arith_type=Unsigned  n_bits=8  bin_pt=2  align_bp=on  dbl_ovrd=off  block_type=logical
      settings: xl_area=[1 0 0 1 0 0 0]  block_version=VER_STRING_GOES_HERE
  Posedge1 : Subsystem
  Posedge2 : Subsystem
  Relational2 : xbsIndex_r4/Relational  mode=a>=b  en=off  latency=0  dbl_ovrd=off  block_type=relational
  S-R Latch1 : Subsystem
  Timeout Counter : xbsIndex_r4/Counter  cnt_type=Free Running  cnt_to=Inf  operation=Up  start_count=1  cnt_by_val=1  arith_type=Unsigned  n_bits=NB_CNTR_ACKTIMEOUT  bin_pt=0  load_pin=off  rst=on  en=on  explicit_period=off  period=1  dbl_ovrd=off  use_behavioral_HDL=off  implementation=Fabric  block_type=counter
  Timeout Done : Outport
  wires:
  Posedge1/1(Q) -> Timeout Done/1
  Posedge2/1(Q) -> S-R Latch1/1(S)
  [Tx_Ctrl_Timeout_Start] -> Posedge2/1(D)
  Timeout Counter/1 -> Relational2/1
  [reg_Interval_ACK_Timeout] -> Relational2/2
  Relational2/1 -> Posedge1/1(D), Logical2/1, Logical3/3
  Logical2/1 -> Timeout Counter/1
  Inverter/1 -> Logical2/2
  [PHY_RX_START_IND] -> Logical3/1
  Logical3/1 -> S-R Latch1/2(R)
  [GLOBAL_RESET] -> Logical3/2
  S-R Latch1/1(Q) -> Timeout Counter/2, Inverter/1

== system wlan_mac_dcf_hw/Auto Tx Control/Posedge1 ==
  note: Rising Edge Detection
  D : Inport
  Delay : xbsIndex_r4/Delay  rst=off  infoeditControl=Selection of Reset will increase slice count due to use of real FFs and instead of SRLs  en=off  latency=1  dbl_ovrd=off  reg_retiming=off  block_type=delay
      settings: infoedit=Hardware notes: A delay line is a chain, each link of which is an SRL16 followed by a flip-flop. If register retiming is enabled, the delay line is a chain of flip-flops.  xl_area=[1 1 0 0 0 0 0]  block_version=VER_STRING_GOES_HERE
  Inverter : xbsIndex_r4/Inverter  en=off  latency=0  dbl_ovrd=off  block_type=inv
      settings: xl_area=[0 0 0 0 0 0 0]  block_version=VER_STRING_GOES_HERE
  Logical1 : xbsIndex_r4/Logical  logical_function=AND  inputs=2  en=off  latency=0  precision=Full  arith_type=Unsigned  n_bits=8  bin_pt=2  align_bp=on  dbl_ovrd=off  block_type=logical
      settings: xl_area=[1 0 0 1 0 0 0]  block_version=VER_STRING_GOES_HERE
  Q : Outport
  wires:
  Delay/1 -> Inverter/1
  Inverter/1 -> Logical1/1
  Logical1/1 -> Q/1
  D/1 -> Delay/1, Logical1/2

== system wlan_mac_dcf_hw/Auto Tx Control/Posedge2 ==
  note: Rising Edge Detection
  D : Inport
  Delay : xbsIndex_r4/Delay  rst=off  infoeditControl=Selection of Reset will increase slice count due to use of real FFs and instead of SRLs  en=off  latency=1  dbl_ovrd=off  reg_retiming=off  block_type=delay
      settings: infoedit=Hardware notes: A delay line is a chain, each link of which is an SRL16 followed by a flip-flop. If register retiming is enabled, the delay line is a chain of flip-flops.  xl_area=[1 1 0 0 0 0 0]  block_version=VER_STRING_GOES_HERE
  Inverter : xbsIndex_r4/Inverter  en=off  latency=0  dbl_ovrd=off  block_type=inv
      settings: xl_area=[0 0 0 0 0 0 0]  block_version=VER_STRING_GOES_HERE
  Logical1 : xbsIndex_r4/Logical  logical_function=AND  inputs=2  en=off  latency=0  precision=Full  arith_type=Unsigned  n_bits=8  bin_pt=2  align_bp=on  dbl_ovrd=off  block_type=logical
      settings: xl_area=[1 0 0 1 0 0 0]  block_version=VER_STRING_GOES_HERE
  Q : Outport
  wires:
  D/1 -> Logical1/2, Delay/1
  Logical1/1 -> Q/1
  Inverter/1 -> Logical1/1
  Delay/1 -> Inverter/1

== system wlan_mac_dcf_hw/Auto Tx Control/S-R Latch1 ==
  S : Inport
  R : Inport  Port=2
  Constant1 : xbsIndex_r4/Constant  const=1  gui_display_data_type=Boolean  arith_type=Boolean  n_bits=1  bin_pt=0  preci_type=Single  exp_width=8  frac_width=24  explicit_period=off  period=1  equ=P=C  opselect=C  inp2=PCIN>>17  opr=+  inp1=P  carry=CIN  dbl_ovrd=off  block_type=constant
      settings: block_version=VER_STRING_GOES_HERE
  Register2 : xbsIndex_r4/Register  init=0  rst=on  en=on  dbl_ovrd=off  block_type=register
      settings: xl_area=[1 1 0 0 0 0 0]  block_version=VER_STRING_GOES_HERE
  Q : Outport
  wires:
  S/1 -> Register2/3
  Register2/1 -> Q/1
  R/1 -> Register2/2
  Constant1/1 -> Register2/1

== system wlan_mac_dcf_hw/Auto Tx Control/S-R Latch2 ==
  S : Inport
  R : Inport  Port=2
  Constant1 : xbsIndex_r4/Constant  const=1  gui_display_data_type=Boolean  arith_type=Boolean  n_bits=1  bin_pt=0  preci_type=Single  exp_width=8  frac_width=24  explicit_period=off  period=1  equ=P=C  opselect=C  inp2=PCIN>>17  opr=+  inp1=P  carry=CIN  dbl_ovrd=off  block_type=constant
      settings: block_version=VER_STRING_GOES_HERE
  Register2 : xbsIndex_r4/Register  init=0  rst=on  en=on  dbl_ovrd=off  block_type=register
      settings: xl_area=[1 1 0 0 0 0 0]  block_version=VER_STRING_GOES_HERE
  Q : Outport
  wires:
  Constant1/1 -> Register2/1
  R/1 -> Register2/2
  Register2/1 -> Q/1
  S/1 -> Register2/3

== system wlan_mac_dcf_hw/Auto Tx Control/negedge ==
  D : Inport
  Delay : xbsIndex_r4/Delay  rst=off  infoeditControl=Selection of Reset will increase slice count due to use of real FFs and instead of SRLs  en=off  latency=1  dbl_ovrd=off  reg_retiming=off  block_type=delay
      settings: infoedit=Hardware notes: A delay line is a chain, each link of which is an SRL16 followed by a flip-flop. If register retiming is enabled, the delay line is a chain of flip-flops.  xl_area=[1 1 0 0 0 0 0]  block_version=VER_STRING_GOES_HERE
  Inverter : xbsIndex_r4/Inverter  en=off  latency=0  dbl_ovrd=off  block_type=inv
      settings: xl_area=[0 0 0 0 0 0 0]  block_version=VER_STRING_GOES_HERE
  Logical1 : xbsIndex_r4/Logical  logical_function=AND  inputs=2  en=off  latency=0  precision=Full  arith_type=Unsigned  n_bits=8  bin_pt=2  align_bp=on  dbl_ovrd=off  block_type=logical
      settings: xl_area=[1 0 0 1 0 0 0]  block_version=VER_STRING_GOES_HERE
  Q : Outport
  wires:
  Delay/1 -> Logical1/1
  Logical1/1 -> Q/1
  D/1 -> Delay/1, Inverter/1
  Inverter/1 -> Logical1/2
